simulink model "HArv6dof"  (R2019a)
settings: Solver=VariableStepAuto  StartTime=0.0  StopTime=10  RelTol=1e-3
model workspace (MAT data in the model file):
  op_trim1 : opcond.OperatingReport (value not decoded)
undefined symbols (not defined in the file): ad, ae, airlib, b, B747, cbar, DT, eqm, fms, GM, gr, hlp, m, S
settings Model: Creator=kumabhi  LastModifiedBy=kumabhi
settings DataIOCC: ExternalInput=getinputstruct(op_trim1)  InitialState=getstatestruct(op_trim1)  LoadExternalInput=on  LoadInitialState=on

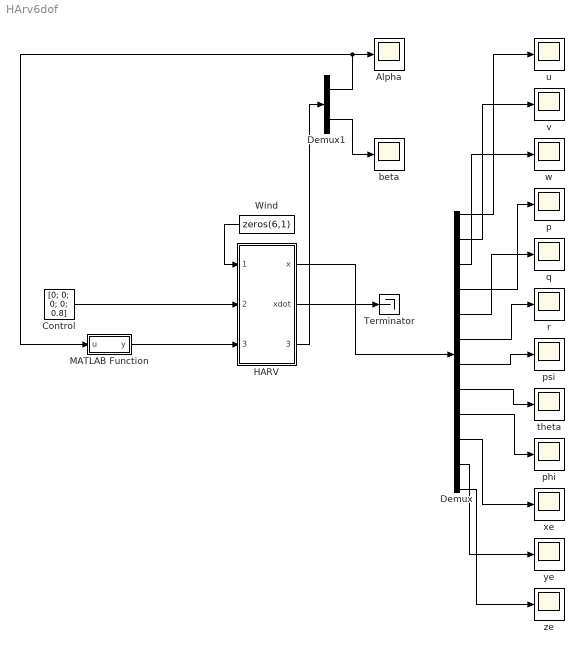
== system HArv6dof ==
  Alpha : Scope
  Control : Constant  Value=[0; 0; 0; 0; 0.8]
  Demux : Demux  Outputs=12
  Demux1 : Demux  Outputs=2
  HARV : Subsystem  AncestorBlock=airlib/DT-B747
  MATLAB Function : MATLAB Function  TreatAsAtomicUnit=on
  Terminator : Terminator
  Wind : Constant  Value=zeros(6,1)
  beta : Scope
  p : Scope
  phi : Scope
  psi : Scope
  q : Scope
  r : Scope
  theta : Scope
  u : Scope
  v : Scope
  w : Scope
  xe : Scope
  ye : Scope
  ze : Scope
  wires:
  HARV/1(x) -> Demux/1
  MATLAB Function/1(y) -> HARV/3(Stability Derivatives)
  Wind/1 -> HARV/1(Wind)
  Control/1 -> HARV/2(Control)
  Demux/1 -> u/1
  Demux/2 -> v/1
  Demux/3 -> w/1
  Demux/4 -> p/1
  Demux/5 -> q/1
  Demux/6 -> r/1
  Demux/7 -> psi/1
  Demux/8 -> theta/1
  Demux/11 -> ye/1
  Demux/12 -> ze/1
  Demux/9 -> phi/1
  Demux/10 -> xe/1
  HARV/3(Yangles) -> Demux1/1
  Demux1/1 -> MATLAB Function/1(u), Alpha/1
  Demux1/2 -> beta/1
  HARV/2(xdot) -> Terminator/1

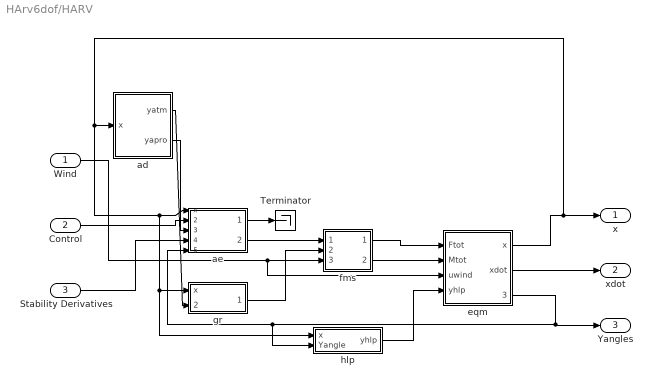
== system HArv6dof/HARV ==
  Wind : Inport
  Control : Inport  Port=2
  Stability Derivatives : Inport  Port=3
  Terminator : Terminator
  ad : Subsystem  AncestorBlock=airlib/DT-B747/ad
  ae : Subsystem  AncestorBlock=airlib/DT-B747/ae
      mask Display: disp('Faero')
  eqm : Subsystem  AncestorBlock=airlib/DT-B747/eqm
  fms : Subsystem  AncestorBlock=airlib/DT-B747/fms  mask(FMsort){}
      mask help: Forces and Moments sorting block
      mask Display: disp('FMsort')
  gr : Subsystem  AncestorBlock=airlib/DT-B747/gr  mask(Gravity){m=m}
      mask prompts: m "Mass of the aircraft [kg]:"
      mask help: Gravity forces.
      mask Display: disp('Gravity')
  hlp : Subsystem  AncestorBlock=airlib/DT-B747/hlp  mask(Hlpfcn){}
      mask help: Help sines and cosines
      mask Display: disp('hlpfcn')
  x : Outport
  xdot : Outport  Port=2
  Yangles : Outport  Port=3
  wires:
  ad/2(yapro) -> ae/3(yaprop)
  Control/1 -> ae/2(Control)
  Stability Derivatives/1 -> ae/4(Stability Derivatives)
  ad/1(yatm) -> gr/2(yatm)
  ae/2(FMaero) -> fms/1(FMaero)
  Wind/1 -> eqm/3(uwind), fms/3(Fwind)
  gr/1(Fgrav) -> fms/2(Fgrav)
  ae/1(Caero) -> Terminator/1
  fms/1(Ftot) -> eqm/1(Ftot)
  fms/2(Mtot) -> eqm/2(Mtot)
  hlp/1(yhlp) -> eqm/4(yhlp)
  eqm/1(x) -> hlp/1(x), gr/1(x), ae/1(x), ad/1(x), x/1
  eqm/2(xdot) -> xdot/1
  eqm/3(Yangles) -> hlp/2(Yangle), ae/5(Yangles), Yangles/1

== system HArv6dof/HARV/ad ==
  x : Inport
  ad1 : Subsystem  mask(Airdata1){}
      mask help: Basic airdata variables
      mask Display: disp('Airdata1')
  atm : Subsystem  mask(Atmosph){}
      mask help: Atmosphere variables
      mask Display: disp('Atmosph')
  yatm : Outport
  yapro : Outport  Port=2
  wires:
  ad1/1(yap) -> yapro/1
  atm/1(yatm) -> ad1/2(yatm), yatm/1
  x/1 -> ad1/1(x), atm/1(x)

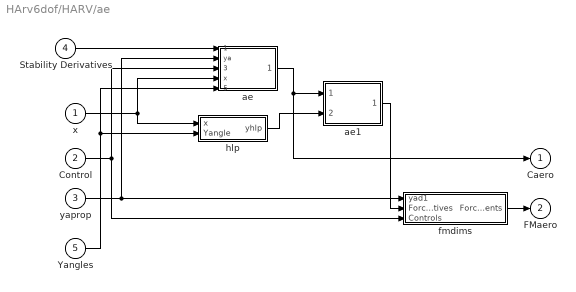
== system HArv6dof/HARV/ae ==
  x : Inport
  Control : Inport  Port=2
  yaprop : Inport  Port=3
  Stability Derivatives : Inport  Port=4
  Yangles : Inport  Port=5
  ae : Subsystem  AncestorBlock=airlib/DT-B747/ae
  ae1 : Subsystem  AncestorBlock=airlib/DT-B747/ae
  fmdims : Subsystem
      mask Display: disp('Forces & Moments')
  hlp : Subsystem  AncestorBlock=airlib/DT-B747/hlp  mask(Hlpfcn){}
      mask help: Help sines and cosines
      mask Display: disp('hlpfcn')
  Caero : Outport
  FMaero : Outport  Port=2
  wires:
  fmdims/1(Forces and moments) -> FMaero/1
  yaprop/1 -> ae/2(ya), fmdims/1(yad1)
  Control/1 -> fmdims/3(Controls), ae/3(Controls)
  Stability Derivatives/1 -> ae/1(Stability Derivatives)
  x/1 -> hlp/1(x), ae/4(x)
  ae/1(Output) -> ae1/1(Caero), Caero/1
  hlp/1(yhlp) -> ae1/2(helpfcn)
  ae1/1(CForce) -> fmdims/2(Force / moment derivatives)
  Yangles/1 -> hlp/2(Yangle), ae/5(Yangles)

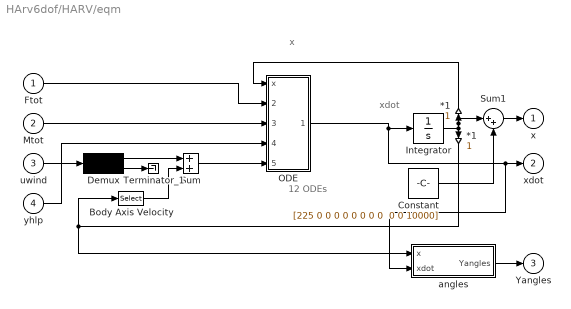
== system HArv6dof/HARV/eqm ==
  note: 12 ODEs
  note: x
  note: xdot
  Ftot : Inport
  Mtot : Inport  Port=2
  uwind : Inport  Port=3
  yhlp : Inport  Port=4
  " *1" : Gain  SaturateOnIntegerOverflow=on  OutDataTypeStr=Inherit: Same as input  ParamDataTypeStr=Inherit: Same as input
  *1 : Gain  SaturateOnIntegerOverflow=on  OutDataTypeStr=Inherit: Same as input  ParamDataTypeStr=Inherit: Same as input
  Body Axis Velocity : Selector  InputPortWidth=12  IndexOptions=Index vector (dialog)  Indices=[1:3]  OutputSizes=1
  Constant : Constant  Value="[225 0 0 0 0 0 0 0 0  0 0 10000]"
  Demux : Demux  Outputs=[3 3]
  Integrator : Integrator  InitialCondition="[225 0 0 0 0 0 0 0 0  0 0 10000]"
  ODE : Subsystem
  Sum : Sum  SaturateOnIntegerOverflow=on  InputSameDT=on  OutDataTypeStr=Inherit: Same as first input
  Sum1 : Sum  Inputs=|++
  Terminator_1 : Terminator
  angles : Subsystem  mask(alpha and beta){}
      mask help: Calculation of alpha and beta
      mask Display: disp('Alpha and Beta')
  x : Outport
  xdot : Outport  Port=2
  Yangles : Outport  Port=3
  wires:
  " *1"/1 -> ODE/1(x)
  ODE/1(xdot) -> Integrator/1, angles/2(xdot), xdot/1
  Integrator/1 -> Sum1/1, *1/1, " *1"/1
  *1/1 -> Body Axis Velocity/1, angles/1(x)
  Mtot/1 -> ODE/3(Mtot)
  Ftot/1 -> ODE/2(Ftot)
  Demux/1 -> Sum/1
  uwind/1 -> Demux/1
  angles/1(Yangles) -> Yangles/1
  Sum/1 -> ODE/5(ybvel*)
  yhlp/1 -> ODE/4(yhlp)
  Demux/2 -> Terminator_1/1
  Body Axis Velocity/1 -> Sum/2
  Constant/1 -> Sum1/2
  Sum1/1 -> x/1

== system HArv6dof/HARV/fms ==
  FMaero : Inport
  Fgrav : Inport  Port=2
  Fwind : Inport  Port=3
  Demux : Demux  Outputs=[3 3]
  Demux1 : Demux  Outputs=[3 3]
  Sum3 : Sum  Inputs=+++  SaturateOnIntegerOverflow=on  InputSameDT=on  OutDataTypeStr=Inherit: Same as first input
  Terminator : Terminator
  Ftot : Outport
  Mtot : Outport  Port=2
  wires:
  Demux/1 -> Sum3/1
  Demux/2 -> Mtot/1
  Sum3/1 -> Ftot/1
  Fgrav/1 -> Sum3/3
  FMaero/1 -> Demux/1
  Fwind/1 -> Demux1/1
  Demux1/1 -> Sum3/2
  Demux1/2 -> Terminator/1

== system HArv6dof/HARV/gr ==
  x : Inport
  yatm : Inport  Port=2
  Mux : Mux  Inputs=3
  Mux1 : Mux  Inputs=[12 5]
  Xgr : Fcn  Expr=-m*u[17]*sin(u[8])
  Ygr : Fcn  Expr=m*u[17]*cos(u[8])*sin(u[9])
  Zgr : Fcn  Expr=m*u[17]*cos(u[8])*cos(u[9])
  Fgrav : Outport
  wires:
  yatm/1 -> Mux1/2
  x/1 -> Mux1/1
  Zgr/1 -> Mux/3
  Mux1/1 -> Zgr/1, Xgr/1, Ygr/1
  Mux/1 -> Fgrav/1
  Ygr/1 -> Mux/2
  Xgr/1 -> Mux/1

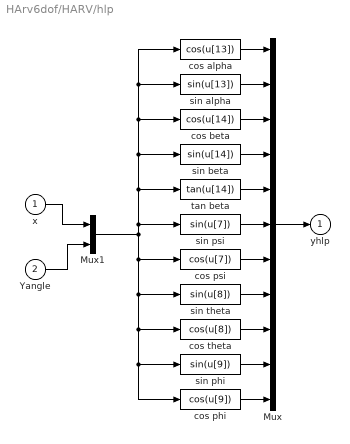
== system HArv6dof/HARV/hlp ==
  x : Inport
  Yangle : Inport  Port=2
  Mux : Mux  Inputs=11
  Mux1 : Mux  Inputs=2
  cos alpha : Fcn  Expr=cos(u[13])
  cos beta : Fcn  Expr=cos(u[14])
  cos phi : Fcn  Expr=cos(u[9])
  cos psi : Fcn  Expr=cos(u[7])
  cos theta : Fcn  Expr=cos(u[8])
  sin alpha : Fcn  Expr=sin(u[13])
  sin beta : Fcn  Expr=sin(u[14])
  sin phi : Fcn  Expr=sin(u[9])
  sin psi : Fcn  Expr=sin(u[7])
  sin theta : Fcn  Expr=sin(u[8])
  tan beta : Fcn  Expr=tan(u[14])
  yhlp : Outport
  wires:
  cos phi/1 -> Mux/11
  Mux/1 -> yhlp/1
  sin phi/1 -> Mux/10
  cos theta/1 -> Mux/9
  sin theta/1 -> Mux/8
  cos psi/1 -> Mux/7
  sin psi/1 -> Mux/6
  tan beta/1 -> Mux/5
  sin beta/1 -> Mux/4
  cos beta/1 -> Mux/3
  sin alpha/1 -> Mux/2
  cos alpha/1 -> Mux/1
  x/1 -> Mux1/1
  Yangle/1 -> Mux1/2
  Mux1/1 -> sin psi/1, tan beta/1, sin beta/1, cos beta/1, sin alpha/1, cos alpha/1, cos phi/1, sin phi/1, cos theta/1, sin theta/1, cos psi/1

== system HArv6dof/HARV/ad/ad1 ==
  x : Inport
  yatm : Inport  Port=2
  M : Fcn  Expr=((u[2]^2+u[3]^2+u[4]^2)^0.5)/u[1]
  Mux : Mux  Inputs=[1 12]
  Mux1 : Mux  Inputs=[12 5]
  Mux2 : Mux  Inputs=3
  a : Fcn  Expr=sqrt(401.8743*u[3])
  qdyn : Fcn  Expr=0.5*u[13]*((u[1]^2+u[2]^2+u[3]^2)^0.5)
  yap : Outport
  wires:
  yatm/1 -> a/1, Mux1/2
  x/1 -> Mux1/1, Mux/2
  Mux/1 -> M/1
  Mux1/1 -> qdyn/1
  M/1 -> Mux2/2
  a/1 -> Mux2/1, Mux/1
  qdyn/1 -> Mux2/3
  Mux2/1 -> yap/1

== system HArv6dof/HARV/ad/atm ==
  x : Inport
  Mux : Mux  Inputs=2
  Mux1 : Mux  Inputs=[2 1]
  Mux2 : Mux  Inputs=5
  Ps : Fcn  Expr=101325*(u[2]/288.15)^(u[1]/1.86584)
  T : Fcn  Expr=288.15 - 0.0065*u[12]
  g : Fcn  Expr=9.80665*(6371020/(6371020+u[12]))^2
  mu : Fcn  Expr=(1.458*10^(-6)*u[2]^1.5)/(u[2]+110.4)
  rho : Fcn  Expr=u[3]/(287.053*u[2])
  yatm : Outport
  wires:
  mu/1 -> Mux2/4
  Mux2/1 -> yatm/1
  Mux1/1 -> rho/1
  rho/1 -> Mux2/1
  g/1 -> Mux2/5, Mux/1
  T/1 -> Mux2/3, Mux/2
  Ps/1 -> Mux2/2, Mux1/2
  Mux/1 -> Ps/1, mu/1, Mux1/1
  x/1 -> g/1, T/1

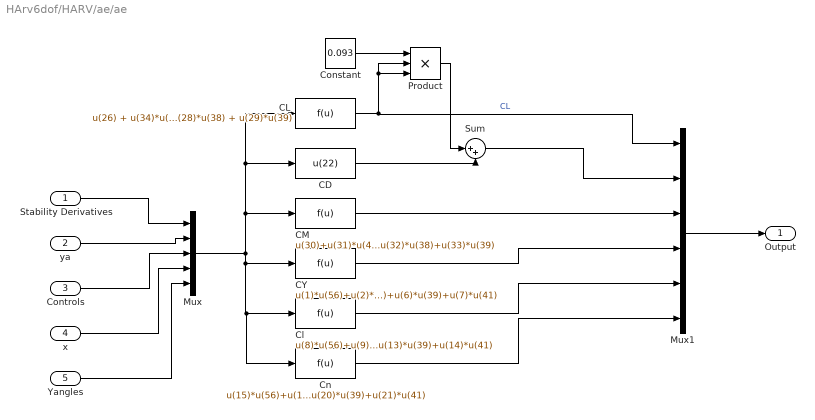
== system HArv6dof/HARV/ae/ae ==
  Stability Derivatives : Inport
  ya : Inport  Port=2
  Controls : Inport  Port=3
  x : Inport  Port=4
  Yangles : Inport  Port=5
  CD : Fcn  Expr=u(22)
  CL : Fcn  Expr=u(26) + u(34)*u(55) + u(27)*u(47)+ u(28)*u(38) + u(29)*u(39)
  CM : Fcn  Expr=u(30)+u(31)*u(47)+u(32)*u(38)+u(33)*u(39)
  CY : Fcn  Expr=u(1)*u(56)+u(2)*u(46)+u(3)*u(48)+u(4)*u(40)+u(5)*u(38)+u(6)*u(39)+u(7)*u(41)
  Cl : Fcn  Expr=u(8)*u(56)+u(9)*u(46)+u(10)*u(48)+u(11)*u(40)+u(12)*u(38)+u(13)*u(39)+u(14)*u(41)
  Cn : Fcn  Expr=u(15)*u(56)+u(16)*u(46)+u(17)*u(48)+u(18)*u(40)+u(19)*u(38)+u(20)*u(39)+u(21)*u(41)
  Constant : Constant  Value=0.093
  Mux : Mux  Inputs=5
  Mux1 : Mux  Inputs=6
  Product : Product  Inputs=3
  Sum : Sum  Inputs=|++
  Output : Outport
  wires:
  Stability Derivatives/1 -> Mux/1
  ya/1 -> Mux/2
  Mux/1 -> CM/1, CD/1, CL/1, Cn/1, Cl/1, CY/1
  Controls/1 -> Mux/3
  x/1 -> Mux/4
  CL/1 -> Product/3, Product/2, Mux1/1  "CL"
  Constant/1 -> Product/1
  Product/1 -> Sum/1
  CD/1 -> Sum/2
  Sum/1 -> Mux1/2
  CM/1 -> Mux1/3
  CY/1 -> Mux1/4
  Cl/1 -> Mux1/5
  Cn/1 -> Mux1/6
  Mux1/1 -> Output/1
  Yangles/1 -> Mux/5

== system HArv6dof/HARV/ae/ae1 ==
  Caero : Inport
  helpfcn : Inport  Port=2
  CX : Fcn  Expr=-u(2)*u(7)+u(1)*u(8)
  CZ : Fcn  Expr=-u(2)*u(8)-u(1)*u(7)
  Demux : Demux
  Mux : Mux  Inputs=2
  Mux1 : Mux  Inputs=6
  Selector : Selector  InputPortWidth=17  IndexOptions=Index vector (dialog)  Indices=[3:6]  OutputSizes=1
  CForce : Outport
  wires:
  Caero/1 -> Mux/1
  helpfcn/1 -> Mux/2
  Mux/1 -> Selector/1, CZ/1, CX/1
  CX/1 -> Mux1/1
  Mux1/1 -> CForce/1
  Selector/1 -> Demux/1
  CZ/1 -> Mux1/3
  Demux/2 -> Mux1/2
  Demux/3 -> Mux1/4
  Demux/1 -> Mux1/5
  Demux/4 -> Mux1/6

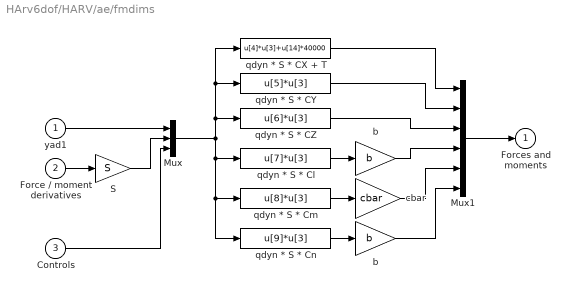
== system HArv6dof/HARV/ae/fmdims ==
  yad1 : Inport
  Force / moment derivatives : Inport  Port=2
  Controls : Inport  Port=3
  Mux : Mux  Inputs=[3 6 5]
  Mux1 : Mux  Inputs=6
  S : Gain  Gain=S  SaturateOnIntegerOverflow=on  OutDataTypeStr=Inherit: Same as input  ParamDataTypeStr=Inherit: Same as input
  b : Gain  Gain=b  SaturateOnIntegerOverflow=on  OutDataTypeStr=Inherit: Same as input  ParamDataTypeStr=Inherit: Same as input
  "b " : Gain  Gain=b  SaturateOnIntegerOverflow=on  OutDataTypeStr=Inherit: Same as input  ParamDataTypeStr=Inherit: Same as input
  cbar : Gain  Gain=cbar  SaturateOnIntegerOverflow=on  OutDataTypeStr=Inherit: Same as input  ParamDataTypeStr=Inherit: Same as input
  qdyn * S * CX + T : Fcn  Expr=u[4]*u[3]+u[14]*40000
  qdyn * S * CY : Fcn  Expr=u[5]*u[3]
  qdyn * S * CZ : Fcn  Expr=u[6]*u[3]
  qdyn * S * Cl : Fcn  Expr=u[7]*u[3]
  qdyn * S * Cm : Fcn  Expr=u[8]*u[3]
  qdyn * S * Cn : Fcn  Expr=u[9]*u[3]
  Forces and moments : Outport
  wires:
  b/1 -> Mux1/4
  qdyn * S * CZ/1 -> Mux1/3
  S/1 -> Mux/2
  qdyn * S * CY/1 -> Mux1/2
  qdyn * S * CX + T/1 -> Mux1/1
  yad1/1 -> Mux/1
  qdyn * S * Cn/1 -> "b "/1
  qdyn * S * Cm/1 -> cbar/1
  qdyn * S * Cl/1 -> b/1
  Mux/1 -> qdyn * S * Cn/1, qdyn * S * Cm/1, qdyn * S * Cl/1, qdyn * S * CY/1, qdyn * S * CX + T/1, qdyn * S * CZ/1
  Force / moment derivatives/1 -> S/1
  cbar/1 -> Mux1/5
  "b "/1 -> Mux1/6
  Mux1/1 -> Forces and moments/1
  Controls/1 -> Mux/3

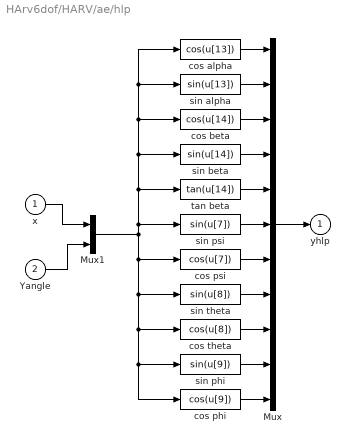
== system HArv6dof/HARV/ae/hlp ==
  x : Inport
  Yangle : Inport  Port=2
  Mux : Mux  Inputs=11
  Mux1 : Mux  Inputs=2
  cos alpha : Fcn  Expr=cos(u[13])
  cos beta : Fcn  Expr=cos(u[14])
  cos phi : Fcn  Expr=cos(u[9])
  cos psi : Fcn  Expr=cos(u[7])
  cos theta : Fcn  Expr=cos(u[8])
  sin alpha : Fcn  Expr=sin(u[13])
  sin beta : Fcn  Expr=sin(u[14])
  sin phi : Fcn  Expr=sin(u[9])
  sin psi : Fcn  Expr=sin(u[7])
  sin theta : Fcn  Expr=sin(u[8])
  tan beta : Fcn  Expr=tan(u[14])
  yhlp : Outport
  wires:
  cos phi/1 -> Mux/11
  Mux/1 -> yhlp/1
  sin phi/1 -> Mux/10
  cos theta/1 -> Mux/9
  sin theta/1 -> Mux/8
  cos psi/1 -> Mux/7
  sin psi/1 -> Mux/6
  tan beta/1 -> Mux/5
  sin beta/1 -> Mux/4
  cos beta/1 -> Mux/3
  sin alpha/1 -> Mux/2
  cos alpha/1 -> Mux/1
  x/1 -> Mux1/1
  Yangle/1 -> Mux1/2
  Mux1/1 -> sin psi/1, tan beta/1, sin beta/1, cos beta/1, sin alpha/1, cos alpha/1, cos phi/1, sin phi/1, cos theta/1, sin theta/1, cos psi/1

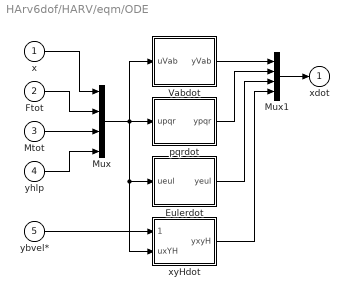
== system HArv6dof/HARV/eqm/ODE ==
  x : Inport
  Ftot : Inport  Port=2
  Mtot : Inport  Port=3
  yhlp : Inport  Port=4
  ybvel* : Inport  Port=5
  Eulerdot : Subsystem  mask(Eulerdot){}
      mask help:
      | Calculation of d(psi)/dt, d(theta)/dt,
      | and d(phi/dt)
      mask Display: disp('psi dot\ntheta dot\nphi dot')
  Mux : Mux  Inputs=[12 3 3 11]
  Mux1 : Mux  Inputs=[3 3 3 3]
  Vabdot : Subsystem  mask(Vabdot){}
      mask help: Calculation of dV/dt, dalpha/dt, dbeta/dt.
      mask Display: disp('u dot\nv dot\nw dot')
  pqrdot : Subsystem  mask(pqrdot){}
      mask help: Calculation of dp/dt, dq/dt, and dr/dt
      mask Display: disp('p dot\nq dot\nr dot')
  xyHdot : Subsystem  mask(xyHdot){}
      mask help: Calculation of d(xe)/dt, d(ye)/dt, and dH/dt
      mask Display: disp('xe dot\nye dot\nH dot')
  xdot : Outport
  wires:
  Mux1/1 -> xdot/1
  Vabdot/1(yVab) -> Mux1/1
  pqrdot/1(ypqr) -> Mux1/2
  Eulerdot/1(yeul) -> Mux1/3
  xyHdot/1(yxyH) -> Mux1/4
  yhlp/1 -> Mux/4
  ybvel*/1 -> xyHdot/1(ybvel*)
  Mux/1 -> xyHdot/2(uxYH), Eulerdot/1(ueul), Vabdot/1(uVab), pqrdot/1(upqr)
  Ftot/1 -> Mux/2
  Mtot/1 -> Mux/3
  x/1 -> Mux/1

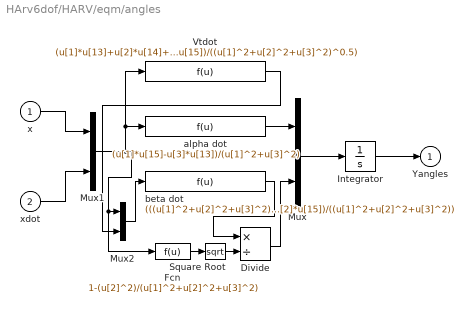
== system HArv6dof/HARV/eqm/angles ==
  x : Inport
  xdot : Inport  Port=2
  Divide : Product  Inputs=*/
  Fcn : Fcn  Expr=1-(u[2]^2)/(u[1]^2+u[2]^2+u[3]^2)
  Integrator : Integrator
  Mux : Mux  Inputs=2
  Mux1 : Mux  Inputs=2
  Mux2 : Mux  Inputs=2
  Square Root : Sqrt  SaturateOnIntegerOverflow=on
  Vtdot : Fcn  Expr=(u[1]*u[13]+u[2]*u[14]+u[3]*u[15])/((u[1]^2+u[2]^2+u[3]^2)^0.5)
  alpha dot : Fcn  Expr=(u[1]*u[15]-u[3]*u[13])/(u[1]^2+u[3]^2)
  beta dot : Fcn  Expr=(((u[1]^2+u[2]^2+u[3]^2)^0.5)*u[14]-u[2]*u[15])/((u[1]^2+u[2]^2+u[3]^2))
  Yangles : Outport
  wires:
  Mux/1 -> Integrator/1
  Mux1/1 -> Vtdot/1, alpha dot/1, Fcn/1, Mux2/1
  beta dot/1 -> Divide/1
  alpha dot/1 -> Mux/1
  x/1 -> Mux1/1
  xdot/1 -> Mux1/2
  Mux2/1 -> beta dot/1
  Vtdot/1 -> Mux2/2
  Integrator/1 -> Yangles/1
  Fcn/1 -> Square Root/1
  Square Root/1 -> Divide/2
  Divide/1 -> Mux/2

== system HArv6dof/HARV/eqm/ODE/Eulerdot ==
  note: yeul=[psi dot; theta dot; phi dot]
  note: ueul=[x;Ftot;Mtot;yhlp]
  ueul : Inport
  Mux1 : Mux  Inputs=[29 1]
  Mux2 : Mux  Inputs=3
  phi dot : Fcn  Expr=u[4] + u[30]*u[26]
  psi dot : Fcn  Expr=(u[5]*u[28] + u[6]*u[29])/u[27]
  theta dot : Fcn  Expr=u[5]*u[29] - u[6]*u[28]
  yeul : Outport
  wires:
  Mux1/1 -> phi dot/1
  phi dot/1 -> Mux2/3
  Mux2/1 -> yeul/1
  theta dot/1 -> Mux2/2
  psi dot/1 -> Mux1/2, Mux2/1
  ueul/1 -> psi dot/1, Mux1/1, theta dot/1

== system HArv6dof/HARV/eqm/ODE/Vabdot ==
  note: uVab=[x;Ftot;Mtot;yhlp]
  note: yVab=[u dot;v dot;w dot]
  uVab : Inport
  Display : Display
  Mux2 : Mux  Inputs=3
  u dot : Fcn  Expr=u[6]*u[2]-u[5]*u[3]+u[13]/m
  v dot : Fcn  Expr=u[4]*u[3]-u[6]*u[1]+u[14]/m
  w dot : Fcn  Expr=u[5]*u[1]-u[4]*u[2]+u[15]/m
  yVab : Outport
  wires:
  uVab/1 -> u dot/1, w dot/1, v dot/1
  v dot/1 -> Mux2/2
  u dot/1 -> Mux2/1
  w dot/1 -> Mux2/3
  Mux2/1 -> Display/1, yVab/1

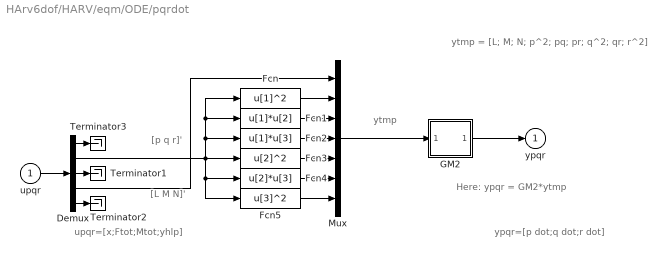
== system HArv6dof/HARV/eqm/ODE/pqrdot ==
  note: [p q r]'
  note: [L M N]'
  note: Here: ypqr = GM2*ytmp
  note: ytmp
  note: ypqr=[p dot;q dot;r dot]
  note: upqr=[x;Ftot;Mtot;yhlp]
  note: ytmp = [L; M; N; p^2; pq; pr; q^2; qr; r^2]
  upqr : Inport
  Demux : Demux  Outputs=[3 3 9 3 11]
  Fcn : Fcn  Expr=u[1]^2
  Fcn1 : Fcn  Expr=u[1]*u[2]
  Fcn2 : Fcn  Expr=u[1]*u[3]
  Fcn3 : Fcn  Expr=u[2]^2
  Fcn4 : Fcn  Expr=u[2]*u[3]
  Fcn5 : Fcn  Expr=u[3]^2
  "GM2 " : Subsystem  mask(State Space){M=GM}
      mask prompts: M "Matrix"
      mask Display: disp('Matrix\nGain')
  Mux : Mux  Inputs=[3 1 1 1 1 1 1]
  Terminator1 : Terminator
  Terminator2 : Terminator
  Terminator3 : Terminator
  ypqr : Outport
  wires:
  upqr/1 -> Demux/1
  Demux/1 -> Terminator3/1
  Demux/5 -> Terminator2/1
  Demux/3 -> Terminator1/1
  Demux/2 -> Fcn1/1, Fcn/1, Fcn2/1, Fcn4/1, Fcn5/1, Fcn3/1
  Demux/4 -> Mux/1
  Fcn/1 -> Mux/2
  Fcn1/1 -> Mux/3
  Fcn2/1 -> Mux/4
  Fcn3/1 -> Mux/5
  Fcn4/1 -> Mux/6
  Fcn5/1 -> Mux/7
  "GM2 "/1(Out1) -> ypqr/1
  Mux/1 -> "GM2 "/1(In1)

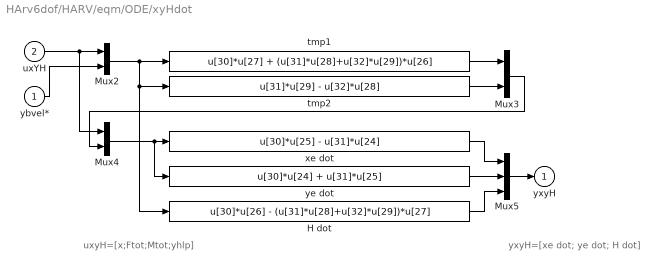
== system HArv6dof/HARV/eqm/ODE/xyHdot ==
  note: yxyH=[xe dot; ye dot; H dot]
  note: uxyH=[x;Ftot;Mtot;yhlp]
  ybvel* : Inport
  uxYH : Inport  Port=2
  H dot : Fcn  Expr=u[30]*u[26] - (u[31]*u[28]+u[32]*u[29])*u[27]
  Mux2 : Mux  Inputs=[29 3]
  Mux3 : Mux  Inputs=2
  Mux4 : Mux  Inputs=[29 2]
  Mux5 : Mux  Inputs=3
  tmp1 : Fcn  Expr=u[30]*u[27] + (u[31]*u[28]+u[32]*u[29])*u[26]
  tmp2 : Fcn  Expr=u[31]*u[29] - u[32]*u[28]
  xe dot : Fcn  Expr=u[30]*u[25] - u[31]*u[24]
  ye dot : Fcn  Expr=u[30]*u[24] + u[31]*u[25]
  yxyH : Outport
  wires:
  tmp1/1 -> Mux3/1
  H dot/1 -> Mux5/3
  xe dot/1 -> Mux5/1
  tmp2/1 -> Mux3/2
  ye dot/1 -> Mux5/2
  Mux5/1 -> yxyH/1
  Mux4/1 -> ye dot/1, xe dot/1
  Mux2/1 -> H dot/1, tmp2/1, tmp1/1
  Mux3/1 -> Mux4/2
  ybvel*/1 -> Mux2/2
  uxYH/1 -> Mux4/1, Mux2/1

== system HArv6dof/HARV/eqm/ODE/pqrdot/GM2  ==
  In1 : Inport
  Matrix Gain : StateSpace  A=[]  B=[]  C=[]  D=GM  InitialCondition=0
  Out1 : Outport
  wires:
  Matrix Gain/1 -> Out1/1
  In1/1 -> Matrix Gain/1

== matlab function HArv6dof/MATLAB Function ==
  data: u input; y output
function y = fcn(u)

y = aero_lookup(u);
